simulink model "sas"  (R2020a)
settings: Solver=VariableStepAuto  StartTime=0.0  StopTime=10.0  RelTol=1e-3
settings Model: Creator=muham  LastModifiedBy=muham

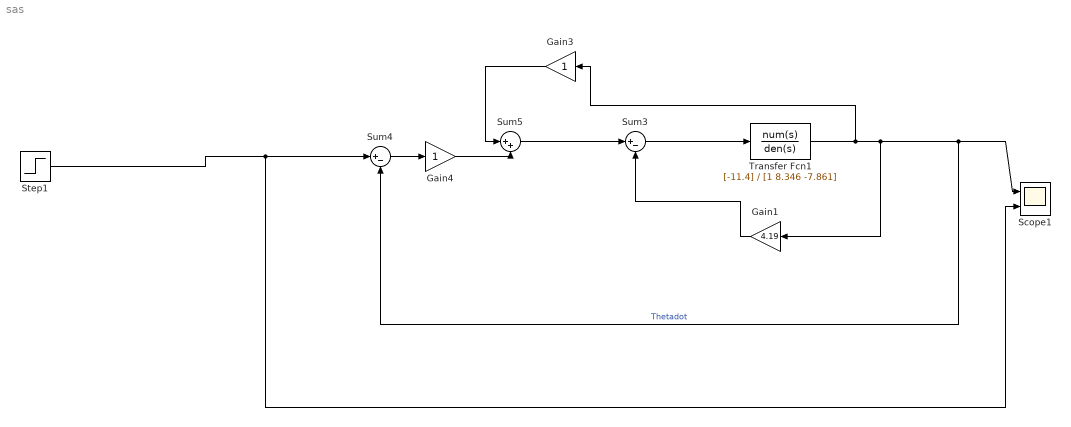
== system sas ==
  Gain1 : Gain  Gain=4.19
  Gain3 : Gain
  Gain4 : Gain
  Scope1 : Scope  NumInputPorts=2
  Step1 : Step  SampleTime=0
  Sum3 : Sum  Inputs=|+-
  Sum4 : Sum  Inputs=|+-
  Sum5 : Sum  Inputs=|++
  Transfer Fcn1 : TransferFcn  Numerator=[-11.4]  Denominator=[1 8.346 -7.861]
  wires:
  Gain4/1 -> Sum5/2
  Sum4/1 -> Gain4/1
  Sum3/1 -> Transfer Fcn1/1
  Gain1/1 -> Sum3/2
  Step1/1 -> Sum4/1, Scope1/2
  Gain3/1 -> Sum5/1
  Transfer Fcn1/1 -> Scope1/1, Sum4/2, Gain1/1, Gain3/1  "Thetadot"
  Sum5/1 -> Sum3/1
